simulink model "simQuad"  (R2016a)
settings: Solver=VariableStepAuto  StartTime=0.0  StopTime=10  FixedStep=dt  RelTol=1e-3
values from neighbouring files (symbols this model uses):
  ic = [-3 0 0 0 0 0 0 0 0 0 0 0]    [cf_pid_compare.m]    (also in main.m = [0 0 0 0 0 0 0 0 0 0 0 0])
  Ki = 0.004    [main.m]
  Kp = 0.5    [main.m]
  r2d = 180/pi    (= 57.2957795131)    [main.m]
  T_takeoff = 5    [main.m]
undefined symbols (not defined in the file or in its folder): default_ctl, run_away
undefined symbols (not defined in the file): cf2, geometric_ctl, ic2
libraries: simulink x22, aerolibtransform2 x10, vrlib x8, aerolibutil x5, cstblocks x4, aerolibnav x2, dspmathops x2
(part 2 of 2)

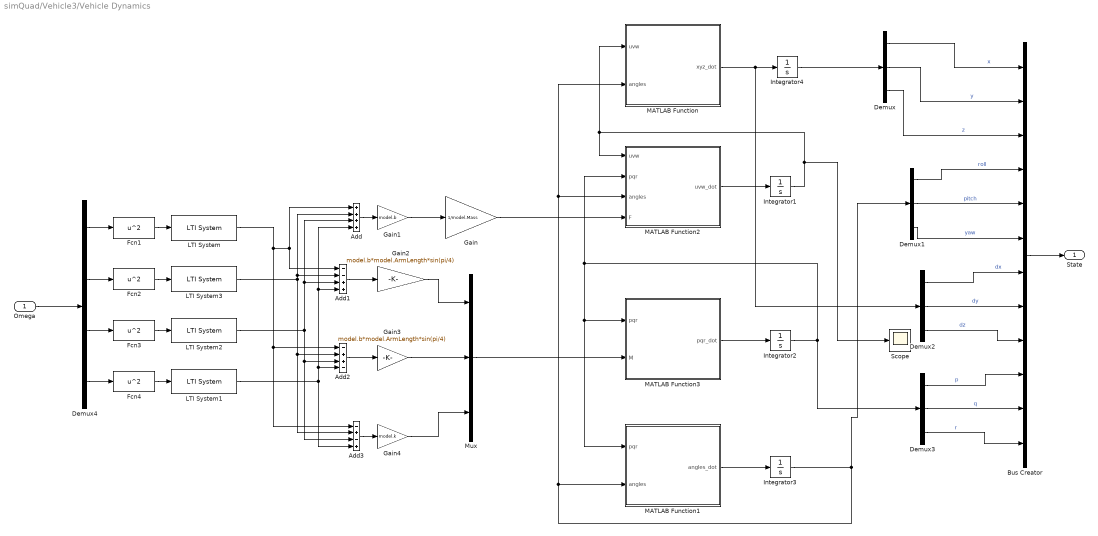
== system simQuad/Vehicle3/Vehicle Dynamics ==
  Omega : Inport
  Add : Sum  Inputs=++++
  Add1 : Sum  Inputs=--++
  Add2 : Sum  Inputs=-++-
  Add3 : Sum  Inputs=-+-+
  Bus Creator : BusCreator  Inputs='x','y','z','roll','pitch','yaw','dx','dy','dz','p','q','r'
  Demux{,1..3} (4 alike) : Demux  Outputs=3
  Demux4 : Demux
  Fcn{1..4} (4 alike) : Fcn  Expr=u^2
  Gain : Gain  Gain=1/model.Mass
  Gain1 : Gain  Gain=model.b
  Gain2 : Gain  Gain=model.b*model.ArmLength*sin(pi/4)
  Gain3 : Gain  Gain=model.b*model.ArmLength*sin(pi/4)
  Gain4 : Gain  Gain=model.k
  Integrator1 : Integrator  InitialCondition=ic(7:9)
  Integrator2 : Integrator  InitialCondition=ic(10:12)
  Integrator3 : Integrator  InitialCondition=ic(4:6)
  Integrator4 : Integrator  InitialCondition=ic(1:3)
  LTI System{,1..3} (4 alike) : cstblocks/LTI System  sys=Gm  IC=[]
  MATLAB Function : MATLAB Function  TreatAsAtomicUnit=on
  MATLAB Function1 : MATLAB Function  TreatAsAtomicUnit=on
  MATLAB Function2 : MATLAB Function  TreatAsAtomicUnit=on
  MATLAB Function3 : MATLAB Function  TreatAsAtomicUnit=on
  Mux : Mux  Inputs=3
  Scope : Scope
  State : Outport
  wires:
  Omega/1 -> Demux4/1
  Demux4/4 -> Fcn4/1
  Demux4/3 -> Fcn3/1
  Demux4/2 -> Fcn2/1
  Demux4/1 -> Fcn1/1
  Demux2/2 -> Bus Creator/8  "dy"
  Demux1/2 -> Bus Creator/5  "pitch"
  Demux3/1 -> Bus Creator/10  "p"
  Demux3/2 -> Bus Creator/11  "q"
  Demux3/3 -> Bus Creator/12  "r"
  Demux2/3 -> Bus Creator/9  "dz"
  Demux2/1 -> Bus Creator/7  "dx"
  Demux1/1 -> Bus Creator/4  "roll"
  Demux1/3 -> Bus Creator/6  "yaw"
  Demux/3 -> Bus Creator/3  "z"
  Demux/2 -> Bus Creator/2  "y"
  Demux/1 -> Bus Creator/1  "x"
  Integrator4/1 -> Demux/1
  Integrator2/1 -> MATLAB Function3/1(pqr), MATLAB Function1/1(pqr), MATLAB Function2/2(pqr), Demux3/1
  Integrator1/1 -> Scope/1, MATLAB Function2/1(uvw), MATLAB Function/1(uvw)
  Integrator3/1 -> MATLAB Function1/2(angles), MATLAB Function2/3(angles), MATLAB Function/2(angles), Demux1/1
  MATLAB Function1/1(angles_dot) -> Integrator3/1
  MATLAB Function3/1(pqr_dot) -> Integrator2/1
  MATLAB Function2/1(uvw_dot) -> Integrator1/1
  MATLAB Function/1(xyz_dot) -> Demux2/1, Integrator4/1
  Mux/1 -> MATLAB Function3/2(M)
  Gain/1 -> MATLAB Function2/4(F)
  Gain3/1 -> Mux/2
  Add3/1 -> Gain4/1
  Gain4/1 -> Mux/3
  Gain2/1 -> Mux/1
  Add2/1 -> Gain3/1
  Add/1 -> Gain1/1
  Add1/1 -> Gain2/1
  Bus Creator/1 -> State/1
  Fcn1/1 -> LTI System/1
  Fcn2/1 -> LTI System3/1
  Fcn3/1 -> LTI System2/1
  Fcn4/1 -> LTI System1/1
  Gain1/1 -> Gain/1
  LTI System1/1 -> Add3/4, Add2/4, Add1/4, Add/4
  LTI System2/1 -> Add3/3, Add2/3, Add/3, Add1/3
  LTI System3/1 -> Add3/2, Add2/2, Add/2, Add1/2
  LTI System/1 -> Add3/1, Add2/1, Add1/1, Add/1

== system simQuad/doest work/DelayStart ==
  In1 : Inport
  Product : Product
  Step : Step  Time=T_takeoff  SampleTime=0
  Out1 : Outport
  wires:
  Step/1 -> Product/1
  Product/1 -> Out1/1
  In1/1 -> Product/2

== system simQuad/doest work/Subsystem ==
  Enable : EnablePort
  Ramp : simulink/Sources/Ramp  slope=1/8  start=0  X0=0
  x* : Sin  Amplitude=0.8  Frequency=2*pi*0.085  Phase=0-0.1  SampleTime=0
  y*1 : Sin  Commented=on  Amplitude=0.8  Frequency=2*pi*0.085  Phase=pi/2-0.1  SampleTime=0
  x : Outport
  y : Outport  Port=2
  wires:
  Ramp/1 -> y/1
  x*/1 -> x/1

== system simQuad/straight line/DelayStart ==
  In1 : Inport
  Product : Product
  Step : Step  Time=T_takeoff  SampleTime=0
  Out1 : Outport
  wires:
  Step/1 -> Product/1
  Product/1 -> Out1/1
  In1/1 -> Product/2

== system simQuad/straight line/Subsystem ==
  Enable : EnablePort
  Ramp : simulink/Sources/Ramp  slope=1/8  start=0  X0=0
  x* : Sin  Amplitude=0.8  Frequency=2*pi*0.085  Phase=0-0.1  SampleTime=0
  y*1 : Sin  Commented=on  Amplitude=0.8  Frequency=2*pi*0.085  Phase=pi/2-0.1  SampleTime=0
  x : Outport
  y : Outport  Port=2
  wires:
  Ramp/1 -> y/1
  x*/1 -> x/1

== system simQuad/straight line/Subsystem1 ==
  In1 : Inport
  Add : Sum
  Ramp : simulink/Sources/Ramp  slope=run_away  start=0  X0=0
  Out1 : Outport
  wires:
  Ramp/1 -> Add/2
  In1/1 -> Add/1
  Add/1 -> Out1/1

== system simQuad/straight line/Subsystem2 ==
  In1 : Inport
  Add : Sum
  Ramp : simulink/Sources/Ramp  slope=run_away  start=0  X0=0
  Out1 : Outport
  wires:
  Add/1 -> Out1/1
  In1/1 -> Add/1
  Ramp/1 -> Add/2

== system simQuad/Controller/Attitude Control/PID ==
  Desired : Inport
  Measured : Inport  Port=2
  Add : Sum  Inputs=3
  Derivative : Derivative
  Integrator Limited : Integrator  LimitOutput=on  UpperSaturationLimit=intSat(2,1)  LowerSaturationLimit=-intSat(2,1)
  Kd : Gain  Gain=att(1,3)  OutMin=[-200]  OutMax=[200]
  Ki : Gain  Gain=att(1,2)  OutMin=[-200]  OutMax=[200]
  Kp : Gain  Gain=att(1,1)  OutMin=[-200]  OutMax=[200]
  Subtract : Sum  Inputs=+-
  Output : Outport
  wires:
  Measured/1 -> Subtract/2
  Desired/1 -> Subtract/1
  Ki/1 -> Add/2
  Add/1 -> Output/1
  Kp/1 -> Add/1
  Kd/1 -> Add/3
  Subtract/1 -> Kp/1, Integrator Limited/1, Derivative/1
  Integrator Limited/1 -> Ki/1
  Derivative/1 -> Kd/1

== system simQuad/Controller/Attitude Control/PID1 ==
  Desired : Inport
  Measured : Inport  Port=2
  Add : Sum  Inputs=3
  Derivative : Derivative
  Integrator Limited1 : Integrator  LimitOutput=on  UpperSaturationLimit=intSat(2,2)  LowerSaturationLimit=-intSat(2,2)
  Kd : Gain  Gain=att(2,3)  OutMin=[-200]  OutMax=[200]
  Ki : Gain  Gain=att(2,2)  OutMin=[-200]  OutMax=[200]
  Kp : Gain  Gain=att(2,1)  OutMin=[-200]  OutMax=[200]
  Subtract : Sum  Inputs=+-
  Output : Outport
  wires:
  Derivative/1 -> Kd/1
  Integrator Limited1/1 -> Ki/1
  Subtract/1 -> Integrator Limited1/1, Derivative/1, Kp/1
  Kd/1 -> Add/3
  Kp/1 -> Add/1
  Add/1 -> Output/1
  Ki/1 -> Add/2
  Desired/1 -> Subtract/1
  Measured/1 -> Subtract/2

== system simQuad/Controller/Attitude Control/PID2 ==
  Desired : Inport
  Measured : Inport  Port=2
  Add : Sum  Inputs=3
  Derivative : Derivative
  Integrator Limited : Integrator  LimitOutput=on  UpperSaturationLimit=intSat(2,3)  LowerSaturationLimit=-intSat(2,3)
  Kd : Gain  Gain=att(3,3)  OutMin=[-200]  OutMax=[200]
  Ki : Gain  Gain=att(3,2)  OutMin=[-200]  OutMax=[200]
  Kp : Gain  Gain=att(3,1)  OutMin=[-200]  OutMax=[200]
  Subtract : Sum  Inputs=+-
  Output : Outport
  wires:
  Measured/1 -> Subtract/2
  Desired/1 -> Subtract/1
  Ki/1 -> Add/2
  Add/1 -> Output/1
  Kp/1 -> Add/1
  Kd/1 -> Add/3
  Subtract/1 -> Kp/1, Integrator Limited/1, Derivative/1
  Integrator Limited/1 -> Ki/1
  Derivative/1 -> Kd/1

== system simQuad/Controller/Linear Velocity Control/PID ==
  Desired : Inport
  Measured : Inport  Port=2
  Add : Sum  Inputs=3
  Derivative : Derivative
  Integrator Limited : Integrator  LimitOutput=on  UpperSaturationLimit=intSat(1,1)  LowerSaturationLimit=-intSat(1,1)
  Kd : Gain  Gain=pos(1,3)  OutMin=[-200]  OutMax=[200]
  Ki : Gain  Gain=pos(1,2)  OutMin=[-200]  OutMax=[200]
  Kp : Gain  Gain=pos(1,1)  OutMin=[-200]  OutMax=[200]
  Subtract : Sum  Inputs=+-
  Output : Outport
  wires:
  Measured/1 -> Subtract/2
  Desired/1 -> Subtract/1
  Ki/1 -> Add/2
  Add/1 -> Output/1
  Kp/1 -> Add/1
  Kd/1 -> Add/3
  Subtract/1 -> Kp/1, Integrator Limited/1, Derivative/1
  Integrator Limited/1 -> Ki/1
  Derivative/1 -> Kd/1

== system simQuad/Controller/Linear Velocity Control/PID1 ==
  Desired : Inport
  Measured : Inport  Port=2
  Add : Sum  Inputs=3
  Derivative : Derivative
  Integrator Limited : Integrator  LimitOutput=on  UpperSaturationLimit=intSat(1,2)  LowerSaturationLimit=-intSat(1,2)
  Kd : Gain  Gain=pos(2,3)  OutMin=[-200]  OutMax=[200]
  Ki : Gain  Gain=pos(2,2)  OutMin=[-200]  OutMax=[200]
  Kp : Gain  Gain=pos(2,1)  OutMin=[-200]  OutMax=[200]
  Subtract : Sum  Inputs=+-
  Output : Outport
  wires:
  Derivative/1 -> Kd/1
  Integrator Limited/1 -> Ki/1
  Subtract/1 -> Derivative/1, Integrator Limited/1, Kp/1
  Kd/1 -> Add/3
  Kp/1 -> Add/1
  Add/1 -> Output/1
  Ki/1 -> Add/2
  Desired/1 -> Subtract/1
  Measured/1 -> Subtract/2

== system simQuad/Controller/Linear Velocity Control/PID_Altitude ==
  z_error : Inport
  Add : Sum  Inputs=3
  Derivative : Derivative
  Integrator Limited : Integrator  LimitOutput=on  UpperSaturationLimit=1000  LowerSaturationLimit=-1000
  Kd : Gain  Gain=pos(3,3)  OutMin=[-200]  OutMax=[200]
  Ki : Gain  Gain=pos(3,2)  OutMin=[-200]  OutMax=[200]
  Kp : Gain  Gain=pos(3,1)  OutMin=[-200]  OutMax=[200]
  Adjust : Outport
  wires:
  Derivative/1 -> Kd/1
  Integrator Limited/1 -> Ki/1
  Kd/1 -> Add/3
  Kp/1 -> Add/1
  Ki/1 -> Add/2
  Add/1 -> Adjust/1
  z_error/1 -> Kp/1, Derivative/1, Integrator Limited/1

== system simQuad/Controller/Rate Control/PID ==
  Desired : Inport
  Measured : Inport  Port=2
  Add : Sum  Inputs=3
  Derivative : Derivative
  Integrator Limited : Integrator  LimitOutput=on  UpperSaturationLimit=intSat(3,1)  LowerSaturationLimit=-intSat(3,1)
  Kd : Gain  Gain=rates(1,3)  OutMin=[-200]  OutMax=[200]
  Ki : Gain  Gain=rates(1,2)  OutMin=[-200]  OutMax=[200]
  Kp : Gain  Gain=rates(1,1)  OutMin=[-200]  OutMax=[200]
  Subtract : Sum  Inputs=+-
  Output : Outport
  wires:
  Measured/1 -> Subtract/2
  Desired/1 -> Subtract/1
  Ki/1 -> Add/2
  Add/1 -> Output/1
  Kp/1 -> Add/1
  Kd/1 -> Add/3
  Subtract/1 -> Kp/1, Integrator Limited/1, Derivative/1
  Integrator Limited/1 -> Ki/1
  Derivative/1 -> Kd/1

== system simQuad/Controller/Rate Control/PID1 ==
  Desired : Inport
  Measured : Inport  Port=2
  Add : Sum  Inputs=3
  Derivative : Derivative
  Integrator Limited : Integrator  LimitOutput=on  UpperSaturationLimit=intSat(3,2)  LowerSaturationLimit=-intSat(3,2)
  Kd : Gain  Gain=rates(2,3)  OutMin=[-200]  OutMax=[200]
  Ki : Gain  Gain=rates(2,2)  OutMin=[-200]  OutMax=[200]
  Kp : Gain  Gain=rates(2,1)  OutMin=[-200]  OutMax=[200]
  Subtract : Sum  Inputs=+-
  Output : Outport
  wires:
  Derivative/1 -> Kd/1
  Integrator Limited/1 -> Ki/1
  Subtract/1 -> Derivative/1, Integrator Limited/1, Kp/1
  Kd/1 -> Add/3
  Kp/1 -> Add/1
  Add/1 -> Output/1
  Ki/1 -> Add/2
  Desired/1 -> Subtract/1
  Measured/1 -> Subtract/2

== system simQuad/Controller/Rate Control/PID2 ==
  Desired : Inport
  Measured : Inport  Port=2
  Add : Sum  Inputs=3
  Derivative : Derivative
  Integrator Limited : Integrator  LimitOutput=on  UpperSaturationLimit=intSat(3,3)  LowerSaturationLimit=-intSat(3,3)
  Kd : Gain  Gain=rates(3,3)  OutMin=[-200]  OutMax=[200]
  Ki : Gain  Gain=rates(3,2)  OutMin=[-200]  OutMax=[200]
  Kp : Gain  Gain=rates(3,1)  OutMin=[-200]  OutMax=[200]
  Subtract : Sum  Inputs=+-
  Output : Outport
  wires:
  Measured/1 -> Subtract/2
  Desired/1 -> Subtract/1
  Ki/1 -> Add/2
  Add/1 -> Output/1
  Kp/1 -> Add/1
  Kd/1 -> Add/3
  Subtract/1 -> Kp/1, Integrator Limited/1, Derivative/1
  Integrator Limited/1 -> Ki/1
  Derivative/1 -> Kd/1

== system simQuad/Controller1/Attitude Control/PID ==
  Desired : Inport
  Measured : Inport  Port=2
  Add : Sum  Inputs=3
  Derivative : Derivative
  Integrator Limited : Integrator  LimitOutput=on  UpperSaturationLimit=intSat(2,1)  LowerSaturationLimit=-intSat(2,1)
  Kd : Gain  Gain=att(1,3)  OutMin=[-200]  OutMax=[200]
  Ki : Gain  Gain=att(1,2)  OutMin=[-200]  OutMax=[200]
  Kp : Gain  Gain=att(1,1)  OutMin=[-200]  OutMax=[200]
  Subtract : Sum  Inputs=+-
  Output : Outport
  wires:
  Measured/1 -> Subtract/2
  Desired/1 -> Subtract/1
  Ki/1 -> Add/2
  Add/1 -> Output/1
  Kp/1 -> Add/1
  Kd/1 -> Add/3
  Subtract/1 -> Kp/1, Integrator Limited/1, Derivative/1
  Integrator Limited/1 -> Ki/1
  Derivative/1 -> Kd/1

== system simQuad/Controller1/Attitude Control/PID1 ==
  Desired : Inport
  Measured : Inport  Port=2
  Add : Sum  Inputs=3
  Derivative : Derivative
  Integrator Limited1 : Integrator  LimitOutput=on  UpperSaturationLimit=intSat(2,2)  LowerSaturationLimit=-intSat(2,2)
  Kd : Gain  Gain=att(2,3)  OutMin=[-200]  OutMax=[200]
  Ki : Gain  Gain=att(2,2)  OutMin=[-200]  OutMax=[200]
  Kp : Gain  Gain=att(2,1)  OutMin=[-200]  OutMax=[200]
  Subtract : Sum  Inputs=+-
  Output : Outport
  wires:
  Derivative/1 -> Kd/1
  Integrator Limited1/1 -> Ki/1
  Subtract/1 -> Integrator Limited1/1, Derivative/1, Kp/1
  Kd/1 -> Add/3
  Kp/1 -> Add/1
  Add/1 -> Output/1
  Ki/1 -> Add/2
  Desired/1 -> Subtract/1
  Measured/1 -> Subtract/2

== system simQuad/Controller1/Attitude Control/PID2 ==
  Desired : Inport
  Measured : Inport  Port=2
  Add : Sum  Inputs=3
  Derivative : Derivative
  Integrator Limited : Integrator  LimitOutput=on  UpperSaturationLimit=intSat(2,3)  LowerSaturationLimit=-intSat(2,3)
  Kd : Gain  Gain=att(3,3)  OutMin=[-200]  OutMax=[200]
  Ki : Gain  Gain=att(3,2)  OutMin=[-200]  OutMax=[200]
  Kp : Gain  Gain=att(3,1)  OutMin=[-200]  OutMax=[200]
  Subtract : Sum  Inputs=+-
  Output : Outport
  wires:
  Measured/1 -> Subtract/2
  Desired/1 -> Subtract/1
  Ki/1 -> Add/2
  Add/1 -> Output/1
  Kp/1 -> Add/1
  Kd/1 -> Add/3
  Subtract/1 -> Kp/1, Integrator Limited/1, Derivative/1
  Integrator Limited/1 -> Ki/1
  Derivative/1 -> Kd/1

== system simQuad/Controller1/Linear Velocity Control/PID ==
  Desired : Inport
  Measured : Inport  Port=2
  Add : Sum  Inputs=3
  Derivative : Derivative
  Integrator Limited : Integrator  LimitOutput=on  UpperSaturationLimit=intSat(1,1)  LowerSaturationLimit=-intSat(1,1)
  Kd : Gain  Gain=pos(1,3)  OutMin=[-200]  OutMax=[200]
  Ki : Gain  Gain=pos(1,2)  OutMin=[-200]  OutMax=[200]
  Kp : Gain  Gain=pos(1,1)  OutMin=[-200]  OutMax=[200]
  Subtract : Sum  Inputs=+-
  Output : Outport
  wires:
  Measured/1 -> Subtract/2
  Desired/1 -> Subtract/1
  Ki/1 -> Add/2
  Add/1 -> Output/1
  Kp/1 -> Add/1
  Kd/1 -> Add/3
  Subtract/1 -> Kp/1, Integrator Limited/1, Derivative/1
  Integrator Limited/1 -> Ki/1
  Derivative/1 -> Kd/1

== system simQuad/Controller1/Linear Velocity Control/PID1 ==
  Desired : Inport
  Measured : Inport  Port=2
  Add : Sum  Inputs=3
  Derivative : Derivative
  Integrator Limited : Integrator  LimitOutput=on  UpperSaturationLimit=intSat(1,2)  LowerSaturationLimit=-intSat(1,2)
  Kd : Gain  Gain=pos(2,3)  OutMin=[-200]  OutMax=[200]
  Ki : Gain  Gain=pos(2,2)  OutMin=[-200]  OutMax=[200]
  Kp : Gain  Gain=pos(2,1)  OutMin=[-200]  OutMax=[200]
  Subtract : Sum  Inputs=+-
  Output : Outport
  wires:
  Derivative/1 -> Kd/1
  Integrator Limited/1 -> Ki/1
  Subtract/1 -> Derivative/1, Integrator Limited/1, Kp/1
  Kd/1 -> Add/3
  Kp/1 -> Add/1
  Add/1 -> Output/1
  Ki/1 -> Add/2
  Desired/1 -> Subtract/1
  Measured/1 -> Subtract/2

== system simQuad/Controller1/Linear Velocity Control/PID_Altitude ==
  z_error : Inport
  Add : Sum  Inputs=3
  Derivative : Derivative
  Integrator Limited : Integrator  LimitOutput=on  UpperSaturationLimit=1000  LowerSaturationLimit=-1000
  Kd : Gain  Gain=pos(3,3)  OutMin=[-200]  OutMax=[200]
  Ki : Gain  Gain=pos(3,2)  OutMin=[-200]  OutMax=[200]
  Kp : Gain  Gain=pos(3,1)  OutMin=[-200]  OutMax=[200]
  Adjust : Outport
  wires:
  Derivative/1 -> Kd/1
  Integrator Limited/1 -> Ki/1
  Kd/1 -> Add/3
  Kp/1 -> Add/1
  Ki/1 -> Add/2
  Add/1 -> Adjust/1
  z_error/1 -> Kp/1, Derivative/1, Integrator Limited/1

== system simQuad/Controller1/Rate Control/PID ==
  Desired : Inport
  Measured : Inport  Port=2
  Add : Sum  Inputs=3
  Derivative : Derivative
  Integrator Limited : Integrator  LimitOutput=on  UpperSaturationLimit=intSat(3,1)  LowerSaturationLimit=-intSat(3,1)
  Kd : Gain  Gain=rates(1,3)  OutMin=[-200]  OutMax=[200]
  Ki : Gain  Gain=rates(1,2)  OutMin=[-200]  OutMax=[200]
  Kp : Gain  Gain=rates(1,1)  OutMin=[-200]  OutMax=[200]
  Subtract : Sum  Inputs=+-
  Output : Outport
  wires:
  Measured/1 -> Subtract/2
  Desired/1 -> Subtract/1
  Ki/1 -> Add/2
  Add/1 -> Output/1
  Kp/1 -> Add/1
  Kd/1 -> Add/3
  Subtract/1 -> Kp/1, Integrator Limited/1, Derivative/1
  Integrator Limited/1 -> Ki/1
  Derivative/1 -> Kd/1

== system simQuad/Controller1/Rate Control/PID1 ==
  Desired : Inport
  Measured : Inport  Port=2
  Add : Sum  Inputs=3
  Derivative : Derivative
  Integrator Limited : Integrator  LimitOutput=on  UpperSaturationLimit=intSat(3,2)  LowerSaturationLimit=-intSat(3,2)
  Kd : Gain  Gain=rates(2,3)  OutMin=[-200]  OutMax=[200]
  Ki : Gain  Gain=rates(2,2)  OutMin=[-200]  OutMax=[200]
  Kp : Gain  Gain=rates(2,1)  OutMin=[-200]  OutMax=[200]
  Subtract : Sum  Inputs=+-
  Output : Outport
  wires:
  Derivative/1 -> Kd/1
  Integrator Limited/1 -> Ki/1
  Subtract/1 -> Derivative/1, Integrator Limited/1, Kp/1
  Kd/1 -> Add/3
  Kp/1 -> Add/1
  Add/1 -> Output/1
  Ki/1 -> Add/2
  Desired/1 -> Subtract/1
  Measured/1 -> Subtract/2

== system simQuad/Controller1/Rate Control/PID2 ==
  Desired : Inport
  Measured : Inport  Port=2
  Add : Sum  Inputs=3
  Derivative : Derivative
  Integrator Limited : Integrator  LimitOutput=on  UpperSaturationLimit=intSat(3,3)  LowerSaturationLimit=-intSat(3,3)
  Kd : Gain  Gain=rates(3,3)  OutMin=[-200]  OutMax=[200]
  Ki : Gain  Gain=rates(3,2)  OutMin=[-200]  OutMax=[200]
  Kp : Gain  Gain=rates(3,1)  OutMin=[-200]  OutMax=[200]
  Subtract : Sum  Inputs=+-
  Output : Outport
  wires:
  Measured/1 -> Subtract/2
  Desired/1 -> Subtract/1
  Ki/1 -> Add/2
  Add/1 -> Output/1
  Kp/1 -> Add/1
  Kd/1 -> Add/3
  Subtract/1 -> Kp/1, Integrator Limited/1, Derivative/1
  Integrator Limited/1 -> Ki/1
  Derivative/1 -> Kd/1

== system simQuad/Estimator/AddNoise1/AddNoise ==
  Signal : Inport
  Add2 : Sum
  Band-Limited White Noise : simulink/Sources/Band-Limited White Noise  Cov=0.00005  Ts=0.1  seed=rng_seed
  +Noise : Outport
  wires:
  Band-Limited White Noise/1 -> Add2/2
  Signal/1 -> Add2/1
  Add2/1 -> +Noise/1

== system simQuad/Estimator/AddNoise1/AddNoise1 ==
  Signal : Inport
  Add2 : Sum
  Band-Limited White Noise : simulink/Sources/Band-Limited White Noise  Cov=0.00005  Ts=0.1  seed=rng_seed
  +Noise : Outport
  wires:
  Add2/1 -> +Noise/1
  Signal/1 -> Add2/1
  Band-Limited White Noise/1 -> Add2/2

== system simQuad/Estimator/AddNoise1/AddNoise2 ==
  Signal : Inport
  Add2 : Sum
  Band-Limited White Noise : simulink/Sources/Band-Limited White Noise  Cov=0.00005  Ts=0.1  seed=rng_seed
  +Noise : Outport
  wires:
  Band-Limited White Noise/1 -> Add2/2
  Signal/1 -> Add2/1
  Add2/1 -> +Noise/1

== system simQuad/Estimator/AddNoise3/AddNoise ==
  Signal : Inport
  Add2 : Sum
  Band-Limited White Noise : simulink/Sources/Band-Limited White Noise  Cov=0.00005  Ts=0.1  seed=rng_seed
  +Noise : Outport
  wires:
  Add2/1 -> +Noise/1
  Signal/1 -> Add2/1
  Band-Limited White Noise/1 -> Add2/2

== system simQuad/Estimator/AddNoise3/AddNoise1 ==
  Signal : Inport
  Add2 : Sum
  Band-Limited White Noise : simulink/Sources/Band-Limited White Noise  Cov=0.00005  Ts=0.1  seed=rng_seed
  +Noise : Outport
  wires:
  Band-Limited White Noise/1 -> Add2/2
  Signal/1 -> Add2/1
  Add2/1 -> +Noise/1

== system simQuad/Estimator/AddNoise3/AddNoise2 ==
  Signal : Inport
  Add2 : Sum
  Band-Limited White Noise : simulink/Sources/Band-Limited White Noise  Cov=0.00005  Ts=0.1  seed=rng_seed
  +Noise : Outport
  wires:
  Add2/1 -> +Noise/1
  Signal/1 -> Add2/1
  Band-Limited White Noise/1 -> Add2/2

== system simQuad/Estimator3/AddNoise1/AddNoise ==
  Signal : Inport
  Add2 : Sum
  Band-Limited White Noise : simulink/Sources/Band-Limited White Noise  Cov=0.00005  Ts=0.1  seed=rng_seed
  +Noise : Outport
  wires:
  Add2/1 -> +Noise/1
  Signal/1 -> Add2/1
  Band-Limited White Noise/1 -> Add2/2

== system simQuad/Estimator3/AddNoise1/AddNoise1 ==
  Signal : Inport
  Add2 : Sum
  Band-Limited White Noise : simulink/Sources/Band-Limited White Noise  Cov=0.00005  Ts=0.1  seed=rng_seed
  +Noise : Outport
  wires:
  Band-Limited White Noise/1 -> Add2/2
  Signal/1 -> Add2/1
  Add2/1 -> +Noise/1

== system simQuad/Estimator3/AddNoise1/AddNoise2 ==
  Signal : Inport
  Add2 : Sum
  Band-Limited White Noise : simulink/Sources/Band-Limited White Noise  Cov=0.00005  Ts=0.1  seed=rng_seed
  +Noise : Outport
  wires:
  Add2/1 -> +Noise/1
  Signal/1 -> Add2/1
  Band-Limited White Noise/1 -> Add2/2

== system simQuad/Estimator3/AddNoise3/AddNoise ==
  Signal : Inport
  Add2 : Sum
  Band-Limited White Noise : simulink/Sources/Band-Limited White Noise  Cov=0.00005  Ts=0.1  seed=rng_seed
  +Noise : Outport
  wires:
  Band-Limited White Noise/1 -> Add2/2
  Signal/1 -> Add2/1
  Add2/1 -> +Noise/1

== system simQuad/Estimator3/AddNoise3/AddNoise1 ==
  Signal : Inport
  Add2 : Sum
  Band-Limited White Noise : simulink/Sources/Band-Limited White Noise  Cov=0.00005  Ts=0.1  seed=rng_seed
  +Noise : Outport
  wires:
  Add2/1 -> +Noise/1
  Signal/1 -> Add2/1
  Band-Limited White Noise/1 -> Add2/2

== system simQuad/Estimator3/AddNoise3/AddNoise2 ==
  Signal : Inport
  Add2 : Sum
  Band-Limited White Noise : simulink/Sources/Band-Limited White Noise  Cov=0.00005  Ts=0.1  seed=rng_seed
  +Noise : Outport
  wires:
  Band-Limited White Noise/1 -> Add2/2
  Signal/1 -> Add2/1
  Add2/1 -> +Noise/1

== matlab function simQuad/Vehicle/Vehicle Dynamics/MATLAB Function ==
  data: uvw input; xyz_dot output; angles input
function xyz_dot  = Position(uvw,angles)
xyz_dot = zeros(3,1);
phi = angles(1); %*pi/180;
theta = angles(2); %*pi/180;
psi = angles(3); %*pi/180;
Tb_o = [cos(theta)*cos(psi)                                cos(theta)*sin(psi)                             -sin(theta)  ;   %BBF > Inertial rotation matrix
        sin(phi)*sin(theta)*cos(psi)-cos(phi)*sin(psi)    sin(phi)*sin(theta)*sin(psi)+cos(phi)*cos(psi)  sin(phi)*cos(theta) ;
        cos(phi)*sin(theta)*cos(psi)+sin(phi)*sin(psi)    cos(phi)*sin(theta)*sin(psi)-sin(phi)*cos(psi)   cos(phi)*cos(theta)];

xyz_dot = (Tb_o')*uvw;
end

== matlab function simQuad/Controller/MATLAB Function1 ==
  data: position input; position_error output; desired_position input
function position_error  = world_error(position,desired_position)
%#Position Error in world Frame
position_error = [0;0;0];


position_error = [desired_position(1)-position(1);...
                  desired_position(2)-position(2);...
                  desired_position(3)-position(3)];

end

== matlab function simQuad/Vehicle/Vehicle Dynamics/MATLAB Function1 ==
  data: pqr input; angles_dot output; angles input
function angles_dot  = Angle(pqr,angles)
angles_dot = zeros(3,1);
phi = angles(1); %*pi/180;
theta = angles(2); %*pi/180;

H = [1    sin(phi)*tan(theta)     cos(phi)*tan(theta)
     0       cos(phi)                 -sin(phi)   
     0       sin(phi)/cos(theta)    cos(phi)/cos(theta)];
angles_dot = H*pqr;
end

== matlab function simQuad/Calc_Omg_des  ==
  data: a_des input; omg_des output; j_des input; yaw_des input; dyaw_des input
function omg_des = fcn(a_des,j_des,yaw_des,dyaw_des)
thrust = a_des+[0 0 9.81]';
thrust_norm = norm(thrust);
z_b = thrust/thrust_norm;
x_w = [cos(yaw_des) sin(yaw_des) 0];
y_b = cross(z_b, x_w);
y_b = y_b/norm(y_b);
x_b = cross(y_b, z_b);

h_w = (j_des - dot(z_b,j_des)*z_b)/thrust_norm;

p = -dot(h_w, y_b);
q = dot(h_w, x_b);
r = dyaw_des*z_b(3);
omg_des = [p q r]';

== matlab function simQuad/Vehicle/Vehicle Dynamics/MATLAB Function2 ==
  data: uvw input; uvw_dot output; pqr input; angles input; F input; model parameter
function uvw_dot  = Forces(uvw,pqr,angles,F,model)
uvw_dot = zeros(3,1);
drag = -uvw .* model.c_drag .* model.AirDensity .* model.a;

Force = [0;0;F]+drag;
g_o = [0;0;-9.81];

phi = angles(1); %*pi/180;
theta = angles(2); %*pi/180;
psi = angles(3); %*pi/180;
Tb_o = [cos(theta)*cos(psi)                                cos(theta)*sin(psi)                             -sin(theta)  ;   %BBF > Inertial rotation matrix
        sin(phi)*sin(theta)*cos(psi)-cos(phi)*sin(psi)    sin(phi)*sin(theta)*sin(psi)+cos(phi)*cos(psi)  sin(phi)*cos(theta) ;
        cos(phi)*sin(theta)*cos(psi)+sin(phi)*sin(psi)    cos(phi)*sin(theta)*sin(psi)-sin(phi)*cos(psi)   cos(phi)*cos(theta)];

uvw_dot = Force + Tb_o*g_o - cross(pqr,uvw);
 
end

== matlab function simQuad/Vehicle/Vehicle Dynamics/MATLAB Function3 ==
  data: pqr_dot output; pqr input; M input
function pqr_dot  = Moments(pqr,M)
pqr_dot = zeros(3,1);
Ixx =  1.395e-05;  %2.3951e-5; %1.39e-05; %2.51943e-5; % % %
Iyy = 1.436e-05; %2.3951e-5; %1.436e-05; % 2.54379e-5; % %         %
Izz =  2.173e-05;  %3.2347e-5; %2.173e-05 ; %4.51407e-5; % %         %;%0.160;
J = diag([Ixx Iyy Izz]);    %   I  Flyer rotational inertia matrix     3x3
pqr_dot = inv(J)*(M-cross(pqr,J*pqr));
end

== matlab function simQuad/Estimator/Mahoney/calc v3 ==
  data: q input; v output
function v = fcn(q)
%#codegen
v = zeros(3,1);
v = [2*(q(2)*q(4) - q(1)*q(3))
         2*(q(1)*q(2) + q(3)*q(4))
         q(1)^2 - q(2)^2 - q(3)^2 + q(4)^2];
end

== matlab function simQuad/Estimator/Mahoney/calc v ==
  data: q input; v output
function v = fcn(q)
%#codegen
v = zeros(3,1);
v = [2*(q(2)*q(4) - q(1)*q(3))
         2*(q(1)*q(2) + q(3)*q(4))
         q(1)^2 - q(2)^2 - q(3)^2 + q(4)^2];
end

== matlab function simQuad/Estimator/Mahoney/quatprod ==
  data: a input; ab output; b input
function ab = quaternProd(a, b)
%QUATERNPROD Calculates the quaternion product
%
%   ab = quaternProd(a, b)
%
%   Calculates the quaternion product of quaternion a and b.
%
%   For more information see:
%   http://www.x-io.co.uk/node/8#quaternions
%
%	Date          Author          Notes
%	27/09/2011    SOH Madgwick    Initial release
    ab = zeros(1,4);
    ab(:,1) = a(:,1).*b(:,1)-a(:,2).*b(:,2)-a(:,3).*b(:,3)-a(:,4).*b(:,4);
    ab(:,2) = a(:,1).*b(:,2)+a(:,2).*b(:,1)+a(:,3).*b(:,4)-a(:,4).*b(:,3);
    ab(:,3) = a(:,1).*b(:,3)-a(:,2).*b(:,4)+a(:,3).*b(:,1)+a(:,4).*b(:,2);
    ab(:,4) = a(:,1).*b(:,4)+a(:,2).*b(:,3)-a(:,3).*b(:,2)+a(:,4).*b(:,1);
end

== matlab function simQuad/Controller1/MATLAB Function1 ==
  data: position input; position_error output; desired_position input
function position_error  = world_error(position,desired_position)
%#Position Error in world Frame
position_error = [0;0;0];


position_error = [desired_position(1)-position(1);...
                  desired_position(2)-position(2);...
                  desired_position(3)-position(3)];

end

== matlab function simQuad/Estimator3/Mahoney/calc v ==
  data: q input; v output
function v = fcn(q)
%#codegen
v = zeros(3,1);
v = [2*(q(2)*q(4) - q(1)*q(3))
         2*(q(1)*q(2) + q(3)*q(4))
         q(1)^2 - q(2)^2 - q(3)^2 + q(4)^2];
end

== matlab function simQuad/Estimator3/Mahoney/calc v3 ==
  data: q input; v output
function v = fcn(q)
%#codegen
v = zeros(3,1);
v = [2*(q(2)*q(4) - q(1)*q(3))
         2*(q(1)*q(2) + q(3)*q(4))
         q(1)^2 - q(2)^2 - q(3)^2 + q(4)^2];
end

== matlab function simQuad/Estimator3/Mahoney/quatprod ==
  data: a input; ab output; b input
function ab = quaternProd(a, b)
%QUATERNPROD Calculates the quaternion product
%
%   ab = quaternProd(a, b)
%
%   Calculates the quaternion product of quaternion a and b.
%
%   For more information see:
%   http://www.x-io.co.uk/node/8#quaternions
%
%	Date          Author          Notes
%	27/09/2011    SOH Madgwick    Initial release
    ab = zeros(1,4);
    ab(:,1) = a(:,1).*b(:,1)-a(:,2).*b(:,2)-a(:,3).*b(:,3)-a(:,4).*b(:,4);
    ab(:,2) = a(:,1).*b(:,2)+a(:,2).*b(:,1)+a(:,3).*b(:,4)-a(:,4).*b(:,3);
    ab(:,3) = a(:,1).*b(:,3)-a(:,2).*b(:,4)+a(:,3).*b(:,1)+a(:,4).*b(:,2);
    ab(:,4) = a(:,1).*b(:,4)+a(:,2).*b(:,3)-a(:,3).*b(:,2)+a(:,4).*b(:,1);
end

== matlab function simQuad/Vehicle3/Vehicle Dynamics/MATLAB Function ==
  data: uvw input; xyz_dot output; angles input
function xyz_dot  = Position(uvw,angles)
xyz_dot = zeros(3,1);
phi = angles(1); %*pi/180;
theta = angles(2); %*pi/180;
psi = angles(3); %*pi/180;
Tb_o = [cos(theta)*cos(psi)                                cos(theta)*sin(psi)                             -sin(theta)  ;   %BBF > Inertial rotation matrix
        sin(phi)*sin(theta)*cos(psi)-cos(phi)*sin(psi)    sin(phi)*sin(theta)*sin(psi)+cos(phi)*cos(psi)  sin(phi)*cos(theta) ;
        cos(phi)*sin(theta)*cos(psi)+sin(phi)*sin(psi)    cos(phi)*sin(theta)*sin(psi)-sin(phi)*cos(psi)   cos(phi)*cos(theta)];

xyz_dot = (Tb_o')*uvw;
end

== matlab function simQuad/Vehicle3/Vehicle Dynamics/MATLAB Function1 ==
  data: pqr input; angles_dot output; angles input
function angles_dot  = Angle(pqr,angles)
angles_dot = zeros(3,1);
phi = angles(1); %*pi/180;
theta = angles(2); %*pi/180;

H = [1    sin(phi)*tan(theta)     cos(phi)*tan(theta)
     0       cos(phi)                 -sin(phi)   
     0       sin(phi)/cos(theta)    cos(phi)/cos(theta)];
angles_dot = H*pqr;
end

== matlab function simQuad/Vehicle3/Vehicle Dynamics/MATLAB Function2 ==
  data: uvw input; uvw_dot output; pqr input; angles input; F input
function uvw_dot  = Forces(uvw,pqr,angles,F)
uvw_dot = zeros(3,1);
Force = [0;0;F];
g_o = [0;0;-9.81];
phi = angles(1); %*pi/180;
theta = angles(2); %*pi/180;
psi = angles(3); %*pi/180;
Tb_o = [cos(theta)*cos(psi)                                cos(theta)*sin(psi)                             -sin(theta)  ;   %BBF > Inertial rotation matrix
        sin(phi)*sin(theta)*cos(psi)-cos(phi)*sin(psi)    sin(phi)*sin(theta)*sin(psi)+cos(phi)*cos(psi)  sin(phi)*cos(theta) ;
        cos(phi)*sin(theta)*cos(psi)+sin(phi)*sin(psi)    cos(phi)*sin(theta)*sin(psi)-sin(phi)*cos(psi)   cos(phi)*cos(theta)];

uvw_dot = Force + Tb_o*g_o - cross(pqr,uvw);

end

== matlab function simQuad/Vehicle3/Vehicle Dynamics/MATLAB Function3 ==
  data: pqr_dot output; pqr input; M input
function pqr_dot  = Moments(pqr,M)
pqr_dot = zeros(3,1);
Ixx =  1.395e-05;  %2.3951e-5; %1.39e-05; %2.51943e-5; % % %
Iyy = 1.436e-05; %2.3951e-5; %1.436e-05; % 2.54379e-5; % %         %
Izz =  2.173e-05;  %3.2347e-5; %2.173e-05 ; %4.51407e-5; % %         %;%0.160;
J = diag([Ixx Iyy Izz]);    %   I  Flyer rotational inertia matrix     3x3
pqr_dot = inv(J)*(M-cross(pqr,J*pqr));
end
